simulink model "BLDC_FOC_Control_1"  (R2024b)
settings: Solver=VariableStepAuto  StartTime=0.0  StopTime=1  RelTol=1e-3
values from neighbouring files (symbols this model uses):
  iref = 70    [Parameters_List.m]
  pole_pair_number = 1    [Parameters_List.m]
  psim = 0.0175    [Parameters_List.m]
  Ts = 1e-4    (= 0.0001)    [Parameters_List.m]
  Tsc = 1e-4    (= 0.0001)    [Parameters_List.m]
  Vdc = 48    [Parameters_List.m]
libraries: fl_lib x23, nesl_utility x15, ee_lib x13, eeBldcCommutationLogic x1, eeGeneralControl x1
settings Model: Creator=subhajitroy005  LastModifiedBy=subhajitroy005

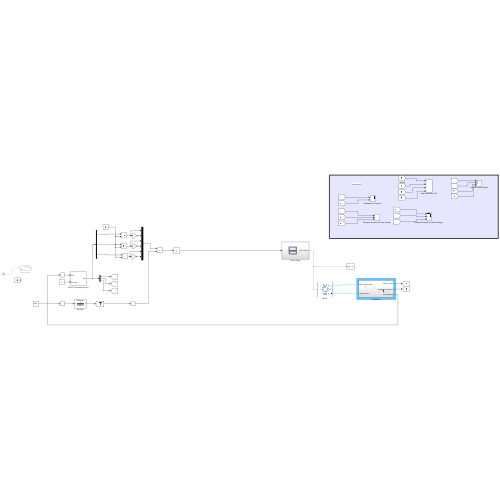
[thumbnail: Simulink's stored preview of the top-level diagram]
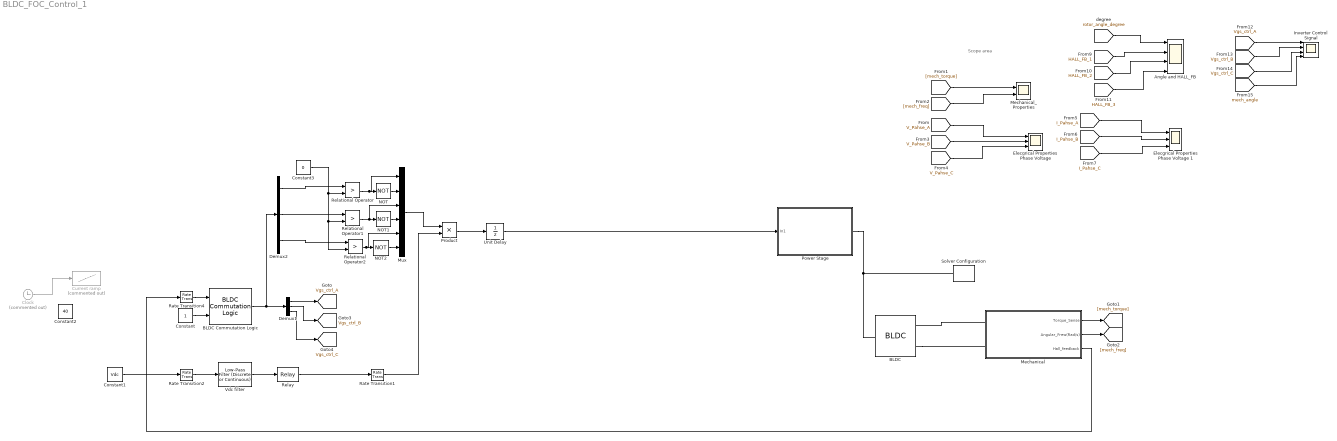
== system BLDC_FOC_Control_1 ==
  note: Scope area
  Angle and HALL_FB : Scope  NumInputPorts=4
  BLDC : ee_lib/Electromechanical/Permanent Magnet/BLDC  port_option=ee.enum.threePhasePort.composite  rotor_param=1  pm_flux_linkage=psim Wb  theta_constant=pi / (2*pole_pair_number) rad  emf_max=9.6 V  w_meas=600 rpm  DphiDtheta_tab=[0, -.1528, -.1528, .1528, .1528, 0] Wb/rad  back_emf_tab=[0, -9.6, -9.6, 9.6, 9.6, 0] V  rotor_angle_tab=[0, 7.5, 22.5, 37.5, 52.5, 60] deg  nPolePairs=pole_pair_number  axes_param=1  winding_type=ee.enum.statorconnection.wye  stator_param=2  machine_param=ee.enum.dqparameterization.constant  Ld=0.00022 H  Lq=0.00022 H  idVec=[-200, 0, 200] A  iqVec=[-200, 0, 200] A  LdMatrix=0.00022 * ones(3, 3) H  LqMatrix=0.00022 * ones(3, 3) H  L0=0.00016 H  Ls=Ls H  Lm=0 H  Ms=Ms H  Rs=Rs Ohm  zero_sequence=ee.enum.park.zerosequence.exclude  loss_param=ee.enum.ironloss.none  losses_oc=[0, 0, 0] W  losses_sc=[0, 0, 0] W  f_losses=60 Hz  Isc_losses=95 A  J=0 kg*m^2  lam=0 N*m/(rad/s)  i_d_specify=on  i_d_priority=High  i_d=0 A  i_d_nominal_specify=off  i_d_nominal_value=1  i_d_nominal_unit=A  i_q_specify=on  i_q_priority=High  i_q=0 A  i_q_nominal_specify=off  i_q_nominal_value=1  i_q_nominal_unit=A  torque_specify=off  torque_priority=None  torque=0 N*m  torque_nominal_specify=off  torque_nominal_value=1  torque_nominal_unit=N*m  angular_velocity_specify=off  angular_velocity_priority=High  angular_velocity=0 rpm  angular_velocity_nominal_specify=off  angular_velocity_nominal_value=1  angular_velocity_nominal_unit=rpm  angular_position_specify=off  angular_position_priority=High  angular_position=0 deg  angular_position_nominal_specify=off  angular_position_nominal_value=1  angular_position_nominal_unit=deg  alpha=3.93e-3 1/K  alpha_flux=-0.001 1/K  Tmeas=298.15 K  stator_thermal_mass=100 J/K  rotor_thermal_mass=200 J/K  Rm_percent_rotor=90  Rd_percent_rotor=30  temperatureA_specify=off  temperatureA_priority=High  temperatureA=25 degC  temperatureA_nominal_specify=off  temperatureA_nominal_value=1  temperatureA_nominal_unit=degC  temperatureB_specify=off  temperatureB_priority=High  temperatureB=25 degC  temperatureB_nominal_specify=off  temperatureB_nominal_value=1  temperatureB_nominal_unit=degC  temperatureC_specify=off  temperatureC_priority=High  temperatureC=25 degC  temperatureC_nominal_specify=off  temperatureC_nominal_value=1  temperatureC_nominal_unit=degC  temperatureR_specify=off  temperatureR_priority=High  temperatureR=25 degC  temperatureR_nominal_specify=off  temperatureR_nominal_value=1  temperatureR_nominal_unit=degC
      settings: InternalSimscapePortConfiguration="{\"Bottom\":[],\"Left\":[{\"id\":\"N\",\"label\":\"~\",\"type\":\"foundation.electrical.three_phase\"}],\"Right\":[{\"id\":\"R\",\"label\":\"R\",\"type\":\"foundation.mechanical.rotational.rotational\"},{\"id\":\"C\",\"label\":\"C\",\"type\":\"foundation.mechanical.rotational.rotational\"}],\"Top\":[]}"
  BLDC Commutation Logic : eeBldcCommutationLogic/BLDC Commutation Logic  Ts=Tsc
  Clock : Clock  Commented=on
  Constant : Constant
  Constant1 : Constant  Value=Vdc  VectorParams1D=off
  Constant2 : Constant  Value=40
  Constant3 : Constant  Value=0
  Current ramp : Lookup_n-D  Commented=on  NumberOfTableDimensions=1  BreakpointsForDimension1=[0 0.5 1]  Table=[0 iref iref]  InternalRulePriority=Speed  RndMeth=Simplest
  Demux1 : Demux  Outputs=3
  Demux2 : Demux  Outputs=3
  "Elecgrical Properties Phase Voltage " : Scope  NumInputPorts=3
  Elecgrical Properties Phase Voltage 1 : Scope  NumInputPorts=3
  Inverter Control Signal : Scope  NumInputPorts=4
  Mechanical : Subsystem
  Mechanical_Properties : Scope  NumInputPorts=2
  Mux : Mux  Inputs=6
  NOT : Logic  Operator=NOT  IconShape=distinctive  AllPortsSameDT=off  OutDataTypeStr=boolean
  NOT1 : Logic  Operator=NOT  IconShape=distinctive  AllPortsSameDT=off  OutDataTypeStr=boolean
  NOT2 : Logic  Operator=NOT  IconShape=distinctive  AllPortsSameDT=off  OutDataTypeStr=boolean
  Power Stage : Subsystem
  Product : Product
  Rate Transition1 : RateTransition  OutPortSampleTime=Ts
  Rate Transition2 : RateTransition  OutPortSampleTime=Tsc
  Rate Transition4 : RateTransition  OutPortSampleTime=Tsc
  Relational Operator : RelationalOperator  Operator=>  OutDataTypeStr=boolean  RndMeth=Simplest  InputSameDT=off
  Relational Operator1 : RelationalOperator  Operator=>  OutDataTypeStr=boolean  RndMeth=Simplest  InputSameDT=off
  Relational Operator2 : RelationalOperator  Operator=>  OutDataTypeStr=boolean  RndMeth=Simplest  InputSameDT=off
  Relay : Relay  OnSwitchValue=Vdc/2  OffSwitchValue=Vdc/4
  Solver Configuration : nesl_utility/Solver Configuration  PhysicalDomain=network_engine_domain  SubClassName=solver  LeftPortType=input  RightPortType=generic  Tones=[]  Harmonics=[]  SimulateNoise=off  Profile=off  UseLocalSampling=off  EnableSwitchedLinearOptims=on  FrequencyDomain=off  UseCCode=off  RelTol=0.001  AbsTol=0.001  MinStep=1e-09  ToWorkspace=off  RevertToSquareIcSolve=off  NumHomotopyIterations=100  PhasorMode=off  PhasorModeNumHarmonics=1  ConsistencySolver=NEWTON_XTOL_AFTER_FTOL  IndexReductionMethod=DerivativeReplacement  DoDC=off  ResidualTolerance=1e-09  ConsistencyTolSource=GLOBAL  ConsistencyAbsTol=0.001  ConsistencyRelTol=0.001  ConsistencyTolFactor=1e-9  UseLocalSolver=on  LocalSolverChoice=NE_BACKWARD_EULER_ADVANCER  ResolveIndetEquations=on  FunctionEvalNumThread=1  LocalSolverSampleTime=Ts  DoFixedCost=on  MaxNonlinIter=5  MaxModeIter=2  ComputeImpulses=off  ImpulseIterations=2  LinearAlgebra=auto  LinearAlgebraNumThread=0  EquationFormulation=NE_TIME_EF  DelaysMemoryBudget=1024  AutomaticFiltering=on  FilteringTimeConstant=0.001  PartitionStorageMethod=AS_NEEDED  PartitionMemoryBudget=1024  PartitionMethod=ROBUST  MultibodyUseLocalSolver=off  MultibodyLocalSolverChoice=ODE1  MultibodyLocalSolverSampleTime=0.001
  Unit Delay : UnitDelay  SampleTime=Ts  HasFrameUpgradeWarning=on
  Vdc filter : eeGeneralControl/Low-Pass Filter (Discrete or Continuous)  K=1  T=0.005  B=inf  A=-inf  init_option=Inherited from block input  x0=0  Ts=Tsc
  tag scope: Vgs_ctrl_A=global, Vgs_ctrl_B=global, Vgs_ctrl_C=global
  wires:
  Clock/1 -> Current ramp/1
  BLDC Commutation Logic/1 -> Demux1/1, Demux2/1
  Rate Transition1/1 -> Product/2
  Relay/1 -> Rate Transition1/1
  Rate Transition4/1 -> BLDC Commutation Logic/1
  Constant/1 -> BLDC Commutation Logic/2
  Rate Transition2/1 -> Vdc filter/1
  Vdc filter/1 -> Relay/1
  Product/1 -> Unit Delay/1
  Mechanical/3(Hall_feedback) -> Rate Transition4/1
  Constant1/1 -> Rate Transition2/1
  Constant3/1 -> Relational Operator2/2, Relational Operator1/2, Relational Operator/2
  Relational Operator/1 -> Mux/1, NOT/1
  Demux2/1 -> Relational Operator/1
  NOT/1 -> Mux/2
  Demux2/2 -> Relational Operator1/1
  NOT1/1 -> Mux/4
  Relational Operator1/1 -> Mux/3, NOT1/1
  Demux2/3 -> Relational Operator2/1
  Relational Operator2/1 -> Mux/5, NOT2/1
  NOT2/1 -> Mux/6
  Mux/1 -> Product/1
  Mechanical/1(Torque_Sense) -> [mech_torque]
  Mechanical/2(Angular_Frew(Rad/s)) -> [mech_freq]
  [mech_freq] -> Mechanical_Properties/2
  [mech_torque] -> Mechanical_Properties/1
  [I_Pahse_A] -> Elecgrical Properties Phase Voltage 1/1
  [I_Pahse_B] -> Elecgrical Properties Phase Voltage 1/2
  [I_Pahse_C] -> Elecgrical Properties Phase Voltage 1/3
  [V_Pahse_A] -> "Elecgrical Properties Phase Voltage "/1
  [V_Pahse_B] -> "Elecgrical Properties Phase Voltage "/2
  [V_Pahse_C] -> "Elecgrical Properties Phase Voltage "/3
  Unit Delay/1 -> Power Stage/1(In1)
  [rotor_angle_degree] -> Angle and HALL_FB/1
  [HALL_FB_1] -> Angle and HALL_FB/2
  [HALL_FB_2] -> Angle and HALL_FB/3
  [HALL_FB_3] -> Angle and HALL_FB/4
  Demux1/1 -> [Vgs_ctrl_A]
  Demux1/2 -> [Vgs_ctrl_B]
  Demux1/3 -> [Vgs_ctrl_C]
  [Vgs_ctrl_A] -> Inverter Control Signal/1
  [Vgs_ctrl_B] -> Inverter Control Signal/2
  [Vgs_ctrl_C] -> Inverter Control Signal/3
  [mech_angle] -> Inverter Control Signal/4
  connections:
  Mechanical/LConn1 -- BLDC/RConn2
  BLDC/RConn1 -- Mechanical/LConn2
  Power Stage/RConn1 -- Solver Configuration/RConn1 -- BLDC/LConn1

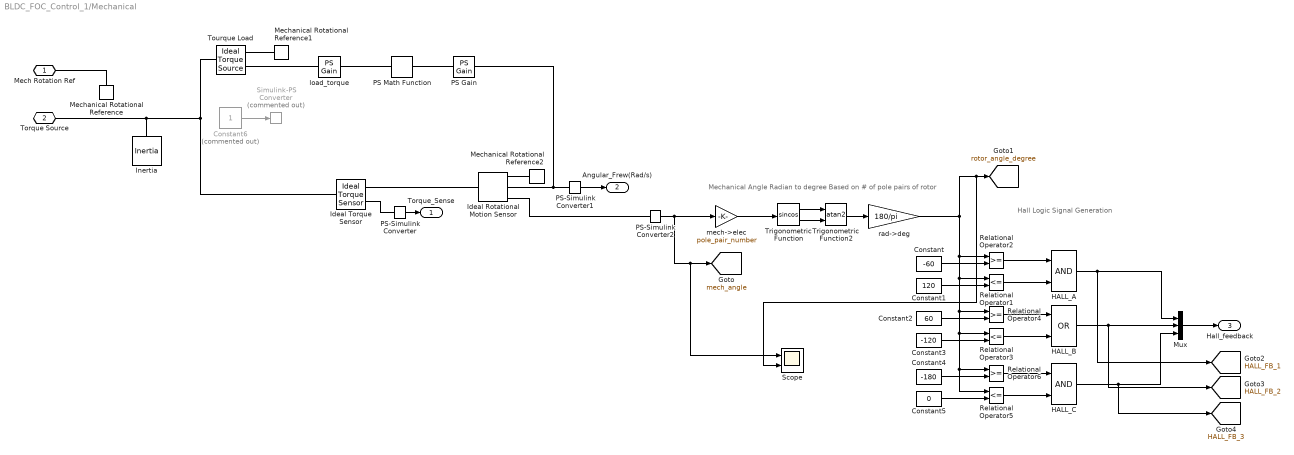
== system BLDC_FOC_Control_1/Mechanical ==
  note: Hall Logic Signal Generation
  note: Mechanical Angle Radian to degree Based on # of pole pairs of rotor
  Constant : Constant  Value=-60
  Constant1 : Constant  Value=120
  Constant2 : Constant  Value=60
  Constant3 : Constant  Value=-120
  Constant4 : Constant  Value=-180
  Constant5 : Constant  Value=0
  Constant6 : Constant  Commented=on
  HALL_A : Logic  AllPortsSameDT=off  OutDataTypeStr=boolean
  HALL_B : Logic  Operator=OR  AllPortsSameDT=off  OutDataTypeStr=boolean
  HALL_C : Logic  AllPortsSameDT=off  OutDataTypeStr=boolean
  Ideal Rotational Motion Sensor : fl_lib/Mechanical/Mechanical Sensors/Ideal Rotational Motion Sensor  reference=foundation.enum.MeasurementReference.difference  acceleration_port=false  velocity_port=true  position_port=true  wrap_angle=true  offset=0 rad
  Ideal Torque Sensor : fl_lib/Mechanical/Mechanical Sensors/Ideal Torque Sensor
  Inertia : fl_lib/Mechanical/Rotational Elements/Inertia  inertia=Jm kg*m^2  num_ports=foundation.enum.numPorts2.one  w_specify=on  w_priority=High  w=0 rad/s  w_nominal_specify=on  w_nominal_value=1  w_nominal_unit=rad/s  t_specify=off  t_priority=None  t=0 N*m  t_nominal_specify=off  t_nominal_value=1  t_nominal_unit=N*m
  Mechanical Rotational Reference : fl_lib/Mechanical/Rotational Elements/Mechanical Rotational Reference
  Mechanical Rotational Reference1 : fl_lib/Mechanical/Rotational Elements/Mechanical Rotational Reference
  Mechanical Rotational Reference2 : fl_lib/Mechanical/Rotational Elements/Mechanical Rotational Reference
  Mux : Mux  Inputs=3
  PS Gain : fl_lib/Physical Signals/Functions/PS Gain  gain=1/200 1/(rad/s)
  PS Math Function : fl_lib/Physical Signals/Functions/PS Math Function  fcn_choice=7  v=1
  PS-Simulink Converter : nesl_utility/PS-Simulink Converter  PhysicalDomain=network_engine_domain  SubClassName=ps_output  LeftPortType=input  RightPortType=output  PseudoPeriodic=off  Frequencies=[]  VectorFormat=inherit  Unit=inherit  AffineConversion=off
  PS-Simulink Converter1 : nesl_utility/PS-Simulink Converter  PhysicalDomain=network_engine_domain  SubClassName=ps_output  LeftPortType=input  RightPortType=output  PseudoPeriodic=off  Frequencies=[]  VectorFormat=inherit  Unit=inherit  AffineConversion=off
  PS-Simulink Converter2 : nesl_utility/PS-Simulink Converter  PhysicalDomain=network_engine_domain  SubClassName=ps_output  LeftPortType=input  RightPortType=output  PseudoPeriodic=off  Frequencies=[]  VectorFormat=inherit  Unit=inherit  AffineConversion=off
  Relational Operator1 : RelationalOperator  Operator=<=
  Relational Operator2 : RelationalOperator
  Relational Operator3 : RelationalOperator  Operator=<=
  Relational Operator4 : RelationalOperator
  Relational Operator5 : RelationalOperator  Operator=<=
  Relational Operator6 : RelationalOperator
  Scope : Scope  NumInputPorts=2
  Simulink-PS Converter : nesl_utility/Simulink-PS Converter  Commented=on  PhysicalDomain=network_engine_domain  SubClassName=ps_input  LeftPortType=input  RightPortType=output  PseudoPeriodic=off  Frequencies=[]  NoiseDistribution=none  NoiseParameters=[]  Unit=1  AffineConversion=off  FilteringAndDerivatives=provide  SimscapeFilterOrder=1  InputFilterTimeConstant=0.001  UdotUserProvided=0
  Tourque Load : fl_lib/Mechanical/Mechanical Sources/Ideal Torque Source
  Trigonometric Function : Trigonometry  Operator=sincos
  Trigonometric Function2 : Trigonometry  Operator=atan2
  load_torque : fl_lib/Physical Signals/Functions/PS Gain  gain=-iref*psim*pole_pair_number*1.5 N*m
  mech->elec : Gain  Gain=pole_pair_number
  rad->deg : Gain  Gain=180/pi  SaturateOnIntegerOverflow=on  OutDataTypeStr=Inherit: Same as input  ParamDataTypeStr=Inherit: Same as input
  Mech Rotation Ref : PMIOPort  Side=Left
  Torque Source : PMIOPort  Port=2  Side=Left
  Torque_Sense : Outport
  Angular_Frew(Rad/s) : Outport  Port=2
  Hall_feedback : Outport  Port=3  VectorParamsAs1DForOutWhenUnconnected=off
  tag scope: HALL_FB_1=global, HALL_FB_2=global, HALL_FB_3=global, mech_angle=global, rotor_angle_degree=global
  wires:
  PS-Simulink Converter/1 -> Torque_Sense/1
  PS-Simulink Converter1/1 -> Angular_Frew(Rad/s)/1
  Trigonometric Function2/1 -> rad->deg/1
  Trigonometric Function/1 -> Trigonometric Function2/1
  mech->elec/1 -> Trigonometric Function/1
  Trigonometric Function/2 -> Trigonometric Function2/2
  Relational Operator5/1 -> HALL_C/2
  Constant2/1 -> Relational Operator4/2
  Relational Operator1/1 -> HALL_A/2
  HALL_B/1 -> [HALL_FB_2], Mux/2
  Relational Operator3/1 -> HALL_B/2
  HALL_C/1 -> [HALL_FB_3], Mux/3
  Relational Operator6/1 -> HALL_C/1
  Constant1/1 -> Relational Operator1/2
  Constant4/1 -> Relational Operator6/2
  Constant3/1 -> Relational Operator3/2
  HALL_A/1 -> Mux/1, [HALL_FB_1]
  Constant/1 -> Relational Operator2/2
  Relational Operator4/1 -> HALL_B/1
  Relational Operator2/1 -> HALL_A/1
  Constant5/1 -> Relational Operator5/2
  Mux/1 -> Hall_feedback/1
  rad->deg/1 -> Scope/2, [rotor_angle_degree], Relational Operator4/1, Relational Operator3/1, Relational Operator5/1, Relational Operator6/1, Relational Operator1/1, Relational Operator2/1
  PS-Simulink Converter2/1 -> Scope/1, [mech_angle], mech->elec/1
  Constant6/1 -> Simulink-PS Converter/1
  connections:
  Tourque Load/LConn1 -- Ideal Torque Sensor/LConn1 -- Torque Source/RConn1 -- Inertia/LConn1
  Mech Rotation Ref/RConn1 -- Mechanical Rotational Reference/LConn1
  Tourque Load/RConn2 -- Mechanical Rotational Reference1/LConn1
  Ideal Rotational Motion Sensor/LConn1 -- Ideal Torque Sensor/RConn1
  Ideal Torque Sensor/RConn2 -- PS-Simulink Converter/LConn1
  Ideal Rotational Motion Sensor/RConn2 -- PS Gain/LConn1 -- PS-Simulink Converter1/LConn1
  Mechanical Rotational Reference2/LConn1 -- Ideal Rotational Motion Sensor/RConn1
  PS-Simulink Converter2/LConn1 -- Ideal Rotational Motion Sensor/RConn3
  PS Gain/RConn1 -- PS Math Function/LConn1
  load_torque/LConn1 -- PS Math Function/RConn1
  load_torque/RConn1 -- Tourque Load/RConn1

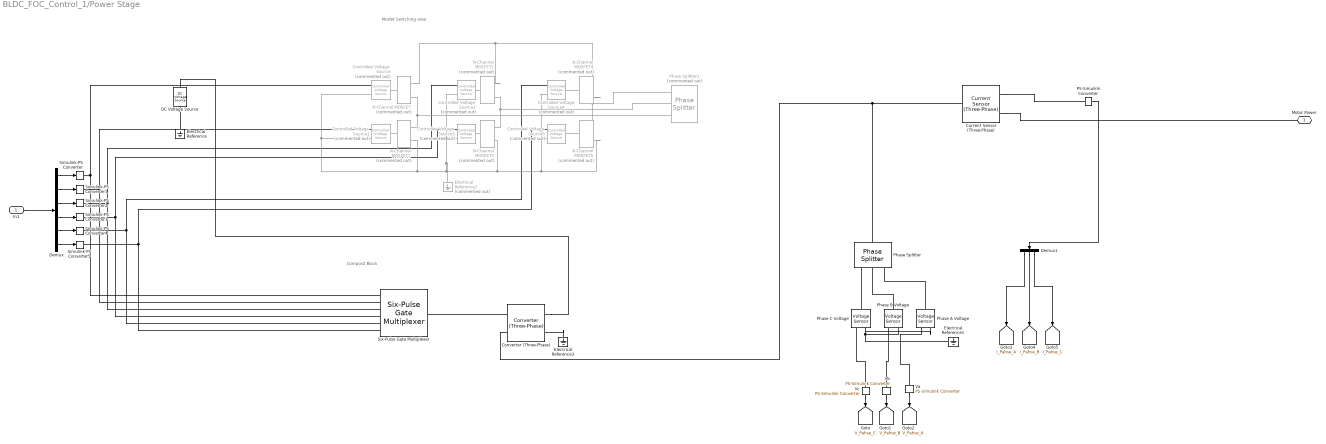
== system BLDC_FOC_Control_1/Power Stage ==
  note: Composit Block
  note: Mosfet Switching area
  In1 : Inport
  Controlled Voltage Source{,1..5} (6 alike) : fl_lib/Electrical/Electrical Sources/Controlled Voltage Source  Commented=on
  Converter (Three-Phase) : ee_lib/Semiconductors & Converters/Converters/Converter (Three-Phase)  port_option=ee.enum.threePhasePort.composite  fidelity_option=ee.enum.converters.fidelity.detailed  device_type=ee.enum.converters.switchingdevice.igbt  showThermalPort=false  K=0  Vth=0.5 V  Vgt=1 V  Vgt_off=-1 V  Ih=1 A  Vf=0.8 V  Ron=0.001 Ohm  Rds=0.001 Ohm  Goff=1e-5 1/Ohm  Eon_scalar=22.86e-3 J  Eoff_scalar=17.14e-3 J  Eoff_natural_commutation=10e-3 J  Voff=300 V  Iout_scalar=600 A  onCurrentMeasDelay=0 s  useCurrentFromPreviousCycle=false  useVoltageFromPreviousCycle=false  diode_param=ee.enum.converters.protectiondiode.nodynamics  diode_Vf=0.8 V  diode_Ron=0.001 Ohm  diode_Goff=1e-5 1/Ohm  diode_C=50 nF  diode_iRM=-235 A  diode_iF=300 A  diode_idot=-50 A/us  diode_trr_param=ee.enum.converters.diodetrr.trr_factor  diode_trr_factor=3  diode_trr=15 us  diode_Qrr=1500 s*uA  diode_rec_loss_model=ee.enum.diode.reverseRecoveryModel.fixed  diode_ErecVal=0 J  diode_scaleWithIandV=false  diode_ErecMat=zeros(2, 3) J  diode_TjrecVec=[298.15, 398.15] K  diode_IfrecVec=[.1, 1, 10] A  diode_IrecVal=10 A  diode_VrecVal=10 V  diode_tFilter=1 / 1000 / 100 s  thermal_network_parameterization=ee.enum.thermalNetworkTopology.external  Rth=[.08, .5] K/W  Rth_Cauer=[.08, .1, .5] K/W  Rth_Foster=[.08, .14, .22, .16] K/W  thermal_mass_parameterization=ee.enum.thermalNetwork.timeconstant  thermal_mass=[.01, .5] J/K  thermal_mass_Cauer=[.01, .1, .5] J/K  thermal_mass_Foster=[.001, .005, .05, .5] J/K  thermal_time_constant=[.001, .2] s  thermal_time_constant_Cauer=[.001, .1, .2] s  thermal_time_constant_Foster=[7e-05, .0007, .01, .08] s  thermal_mass_initial_temperatures=[25, 25] degC  thermal_mass_initial_temperatures_Cauer=[25, 25, 25] degC  junction_thermal_mass=0.01 J/K  Tvec_initial_Foster=[25, 25, 25, 25] degC  snubber_type=ee.enum.converters.snubber.exclude  Cs=1e-7 F  Rs=0.1 Ohm  Vce_loss=[0, 150, 300] V
  Current Sensor (Three-Phase) : ee_lib/Sensors & Transducers/Current Sensor (Three-Phase)
  DC Voltage Source : ee_lib/Additional Components/SPICE Sources/DC Voltage Source  DC=Vdc V
  Demux : Demux  Outputs=6
  Demux1 : Demux  Outputs=3
  Electrical Reference : fl_lib/Electrical/Electrical Elements/Electrical Reference
  Electrical Reference1 : fl_lib/Electrical/Electrical Elements/Electrical Reference
  Electrical Reference2 : fl_lib/Electrical/Electrical Elements/Electrical Reference  Commented=on
  Electrical Reference3 : fl_lib/Electrical/Electrical Elements/Electrical Reference
  N-Channel MOSFET{,1..5} (6 alike) : ee_lib/Semiconductors & Converters/N-Channel MOSFET  Commented=on  paramTerminal=ee.enum.mosfet.numberOfTerminals.three  parameterization=ee.enum.mosfet.parameterization.datasheet  Beta=5.0 A/V^2  Rds=0.025 Ohm  Id=6.0 A  Vgs=5 V  Vth=1.7 V  Vth0=1.7 V  lam=0 1/V  gamma_vth=0.5 V^(1/2)  phib=0.5 V  Vth1=1.9071 V  Vbs1=-1 V  Vth2=2.066 V  Vbs2=-2 V  Tmeas=25 degC  Vgs_vec=[-1, -.5, 2, 3, 4, 5] V  Vds_vec=[0, 2, 4, 8, 12, 16, 20] V  Vbs_vec=[0, -4, -6, -12] V  T_vec=[25, 125] degC  Vth_vec=[.4, 1.2, 1.4, 1.45] V  Vth_mat=[.4, .35; 1.2, 1.15; 1.4, 1.35; 1.45, 1.4] V  Ids_mat=[0, 0, 0, 0, 0, 0, 0; 0, 0, 0, 0, 0, 0, 0; 0, .003, .0038, .0043, .0046, .0048, .0049; 0, .0055, .008, .009, .0095, .01, .0101; 0, .0115, .016, .018, .019, .0195, .02; 0, .0152, .0225, .0265, .028, .0295, .03] A  Ids_mat0=[0, 0, 0, 0, 0, 0, 0; 0, 0, 0, 0, 0, 0, 0; 0, .003, .0038, .0043, .0046, .0048, .0049; 0, .0055, .008, .009, .0095, .01, .0101; 0, .0115, .016, .018, .019, .0195, .02; 0, .0152, .0225, .0265, .028, .0295, .03] A  Ids_mat_3D=zeros(6, 7, 2) A  Ids_mat_3D0=zeros(6, 7, 2) A  IV_table_symmetry=ee.enum.mosfet.symmetricNIV.no  RS=0.0001 Ohm  RD=0.01 Ohm  RB=0.001 Ohm  LeadRs=0 Ohm  LeadRd=0 Ohm  LeadRg=0 Ohm  LeadRb=0 Ohm  LS=0 nH  LD=0 nH  LG=0 nH  LB=0 nH  C_param=ee.enum.mosfet.capacitanceParam.fixedciss  C_GS=270 pF  C_GD=80 pF  C_GB=0 pF  C_DS=0 pF  C_iss=350 pF  C_rss=80 pF  C_oss=0 pF  C_iss_vec=[720, 700, 590, 470, 390, 310] pF  C_rss_vec=[450, 400, 300, 190, 95, 55] pF  C_oss_vec=[900, 810, 690, 420, 270, 170] pF  C_GS_vec=[270, 300, 290, 280, 295, 255] pF  C_GD_vec=[450, 400, 300, 190, 95, 55] pF  C_GB_vec=[270, 300, 290, 280, 295, 255] pF  C_Vgs_vec=0 V  C_DS_vec=[450, 410, 390, 230, 175, 115] pF  C_Vds_vec=[.1, .3, 1, 3, 10, 30] V  V_GS_for_cap_data=0 V  charge_linearity_param=ee.enum.mosfet.cgdLinearity.constant  C_OX=200 pF  V_C_OX=-0.5 V  charge_linearity_param_vgb=ee.enum.mosfet.cgbLinearity.instantly  charge_linearity_param_with_vgb=ee.enum.mosfet.cgbLinearityWithSeparateCgb.instantly  Di_param=ee.enum.mosfet.diodeParam.no  IsDiode=1e-12 A  Vbi=0.6 V  n=1  Cj0Diode=0 pF  TT=50e-9 s  Tmeas_dio=25 degC  TableTypeNoT=ee.enum.mosfet.tableType.IfMat  TableType=ee.enum.diode.tableType.IfMat  IfVec=[.07, .12, .19, 1.75, 4.24, 7.32, 11.2] A  IfMat=[.07, .12, .19, 1.75, 4.24, 7.32, 11.2; .16, .3, .72, 2.14, 4.02, 6.35, 9.12] A  VfVecV=[.9, 1.15, 1.25, 1.5, 1.75, 2.17, 2.6, 2.85] V  VfMatV=[.9, 1.15, 1.25, 1.5, 1.75, 2.17, 2.6, 2.85; .58, .68, .75, 1.1, 1.38, 1.77, 2.27, 2.7] V  TjVec=[25, 125] degC  VfVec=[.5, .7, .9, 1.3, 1.7, 2.1, 2.5] V  IfVecV=[.1, .2, .5, 1, 2, 4, 7, 10] A  diode_Goff=1e-12 1/Ohm  prmDatasheet=ee.enum.temperatureParameterization.none  prmEquCoeff=ee.enum.temperatureParameterization.none  dVth_dT=-6 mV/K  dVth0_dT=-6 mV/K  Rds_T2=0.037 Ohm  BEXDatasheet=-1.5  BEXEquCoeff=-1.5  etaisDatasheet=3  etaisEquCoeff=3  Tmeas2=125 degC  etaisTabulated=3  TdeviceDatasheet=25 degC  TdeviceEquCoeff=25 degC  TdeviceTabulated=25 degC  t_fault=inf s  i_g_specify=off  i_g_priority=None  i_g=0 A  i_g_nominal_specify=off  i_g_nominal_value=1  i_g_nominal_unit=A  i_d_specify=off  i_d_priority=None  i_d=0 A  i_d_nominal_specify=off  i_d_nominal_value=1  i_d_nominal_unit=A  i_b_specify=off  i_b_priority=None  i_b=0 A  i_b_nominal_specify=off  i_b_nominal_value=1  i_b_nominal_unit=A  voltage_gs_specify=off  voltage_gs_priority=None  voltage_gs=0 V  voltage_gs_nominal_specify=off  voltage_gs_nominal_value=1  voltage_gs_nominal_unit=V  voltage_ds_specify=off  voltage_ds_priority=None  voltage_ds=0 V  voltage_ds_nominal_specify=off  voltage_ds_nominal_value=1  voltage_ds_nominal_unit=V  voltage_bs_specify=off  voltage_bs_priority=None  voltage_bs=0 V  voltage_bs_nominal_specify=off  voltage_bs_nominal_value=1  voltage_bs_nominal_unit=V  v_Cgs_specify=off  v_Cgs_priority=High  v_Cgs=0 V  v_Cgs_nominal_specify=off  v_Cgs_nominal_value=1  v_Cgs_nominal_unit=V  v_Cds_specify=off  v_Cds_priority=High  v_Cds=0 V  v_Cds_nominal_specify=off  v_Cds_nominal_value=1  v_Cds_nominal_unit=V  v_Cbs_specify=off  v_Cbs_priority=High  v_Cbs=0 V  v_Cbs_nominal_specify=off  v_Cbs_nominal_value=1  v_Cbs_nominal_unit=V  thermal_network_parameterization=ee.enum.thermalNetworkTopology.junctionCase  Rth=[0, 10] K/W  Rth_Cauer=[1, 3, 10] K/W  Rth_Foster=[.08, .14, .22, .16] K/W  thermal_mass_parameterization=ee.enum.thermalNetwork.timeconstant  thermal_mass=[0, 1] J/K  thermal_mass_Cauer=[.1, .3, 1] J/K  thermal_mass_Foster=[.001, .005, .05, .5] J/K  thermal_time_constant=[0, 10] s  thermal_time_constant_Cauer=[1, 3, 10] s  thermal_time_constant_Foster=[7e-05, .0007, .01, .08] s  thermal_mass_initial_temperatures=[25, 25] degC  thermal_mass_initial_temperatures_Cauer=[25, 25, 25] degC  Tvec_initial_Foster=[25, 25, 25, 25] degC  betaref=18 A/V^2  Vfbref=-1.1 V  gamma=3.5 V^(1/2)  phib2ref=1 V  thesatref=0.4 1/V  alpha=0  Vp=5e-2 V  thesrref=0 1/V  m=8  Tref=25 degC  Rsref=2e-3 Ohm  Rdref=0.17 Ohm  Rgref=8.4 Ohm  Rbref=2e-3 Ohm  Cox=1500 pF  Cgso=100 pF  Cgdo=14 pF  Isref=5.2e-13 A  Cj0=480 pF  Tprm=1  etabet=1.3  Stvfb=5e-4 V/K  Stphib=-8.5e-4 V/K  etasat=1.04  etasr=0.65  etar=0.95  etais=3  Tsim=25 degC  Ig_specify=off  Ig_priority=None  Ig=0 A  Ig_nominal_specify=off  Ig_nominal_value=1  Ig_nominal_unit=A  Ids_specify=off  Ids_priority=None  Ids=0 A  Ids_nominal_specify=off  Ids_nominal_value=1  Ids_nominal_unit=A  Ib_specify=off  Ib_priority=None  Ib=0 A  Ib_nominal_specify=off  Ib_nominal_value=1  Ib_nominal_unit=A  V_gs_specify=off  V_gs_priority=None  V_gs=0 V  V_gs_nominal_specify=off  V_gs_nominal_value=1  V_gs_nominal_unit=V  V_ds_specify=off  V_ds_priority=None  V_ds=0 V  V_ds_nominal_specify=off  V_ds_nominal_value=1  V_ds_nominal_unit=V  V_bs_specify=off  V_bs_priority=None  V_bs=0 V  V_bs_nominal_specify=off  V_bs_nominal_value=1  V_bs_nominal_unit=V  QGoverCox_specify=off  QGoverCox_priority=None  QGoverCox=0 V  QGoverCox_nominal_specify=off  QGoverCox_nominal_value=1  QGoverCox_nominal_unit=V  QDoverCox_specify=off  QDoverCox_priority=None  QDoverCox=0 V  QDoverCox_nominal_specify=off  QDoverCox_nominal_value=1  QDoverCox_nominal_unit=V  QBoverCox_specify=off  QBoverCox_priority=None  QBoverCox=0 V  QBoverCox_nominal_specify=off  QBoverCox_nominal_value=1  QBoverCox_nominal_unit=V  T0=[25, 25] degC  T0_Cauer=[25, 25, 25] degC
  PS-Simulink Converter : nesl_utility/PS-Simulink Converter  PhysicalDomain=network_engine_domain  SubClassName=ps_output  LeftPortType=input  RightPortType=output  PseudoPeriodic=off  Frequencies=[]  VectorFormat=inherit  Unit=inherit  AffineConversion=off
  Phase A Voltage : fl_lib/Electrical/Electrical Sensors/Voltage Sensor
  Phase B Voltage : fl_lib/Electrical/Electrical Sensors/Voltage Sensor
  Phase C Voltage : fl_lib/Electrical/Electrical Sensors/Voltage Sensor
  Phase Splitter : ee_lib/Connectors & References/Phase Splitter
  Phase Splitter2 : ee_lib/Connectors & References/Phase Splitter  Commented=on
  Simulink-PS Converter{,1..5} (6 alike) : nesl_utility/Simulink-PS Converter  PhysicalDomain=network_engine_domain  SubClassName=ps_input  LeftPortType=input  RightPortType=output  PseudoPeriodic=off  Frequencies=[]  NoiseDistribution=none  NoiseParameters=[]  Unit=1  AffineConversion=off  FilteringAndDerivatives=provide  SimscapeFilterOrder=1  InputFilterTimeConstant=0.001  UdotUserProvided=0
  Six-Pulse Gate Multiplexer : ee_lib/Semiconductors & Converters/Converters/Six-Pulse Gate Multiplexer  port_option=ee.enum.controlport.ps
  Va : nesl_utility/PS-Simulink Converter  PhysicalDomain=network_engine_domain  SubClassName=ps_output  LeftPortType=input  RightPortType=output  PseudoPeriodic=off  Frequencies=[]  VectorFormat=inherit  Unit=inherit  AffineConversion=off
  Vb : nesl_utility/PS-Simulink Converter  PhysicalDomain=network_engine_domain  SubClassName=ps_output  LeftPortType=input  RightPortType=output  PseudoPeriodic=off  Frequencies=[]  VectorFormat=inherit  Unit=inherit  AffineConversion=off
  Vc : nesl_utility/PS-Simulink Converter  PhysicalDomain=network_engine_domain  SubClassName=ps_output  LeftPortType=input  RightPortType=output  PseudoPeriodic=off  Frequencies=[]  VectorFormat=inherit  Unit=inherit  AffineConversion=off
  Motor Power : PMIOPort  Side=Right
  tag scope: I_Pahse_A=global, I_Pahse_B=global, I_Pahse_C=global, V_Pahse_A=global, V_Pahse_B=global, V_Pahse_C=global
  wires:
  Demux/1 -> Simulink-PS Converter/1
  Demux/3 -> Simulink-PS Converter2/1
  Demux/2 -> Simulink-PS Converter1/1
  Demux/4 -> Simulink-PS Converter3/1
  Demux/5 -> Simulink-PS Converter4/1
  Demux/6 -> Simulink-PS Converter5/1
  PS-Simulink Converter/1 -> Demux1/1
  In1/1 -> Demux/1
  Demux1/1 -> [I_Pahse_A]
  Demux1/2 -> [I_Pahse_B]
  Demux1/3 -> [I_Pahse_C]
  Vc/1 -> [V_Pahse_C]
  Vb/1 -> [V_Pahse_B]
  Va/1 -> [V_Pahse_A]
  connections:
  Simulink-PS Converter/RConn1 -- Controlled Voltage Source/RConn1 -- Six-Pulse Gate Multiplexer/LConn1
  Simulink-PS Converter2/RConn1 -- Controlled Voltage Source2/RConn1 -- Six-Pulse Gate Multiplexer/LConn3
  Six-Pulse Gate Multiplexer/LConn2 -- Controlled Voltage Source1/RConn1 -- Simulink-PS Converter1/RConn1
  Simulink-PS Converter3/RConn1 -- Controlled Voltage Source3/RConn1 -- Six-Pulse Gate Multiplexer/LConn4
  Simulink-PS Converter4/RConn1 -- Controlled Voltage Source4/RConn1 -- Six-Pulse Gate Multiplexer/LConn5
  Simulink-PS Converter5/RConn1 -- Controlled Voltage Source5/RConn1 -- Six-Pulse Gate Multiplexer/LConn6
  Current Sensor (Three-Phase)/LConn1 -- Converter (Three-Phase)/LConn2 -- Phase Splitter/LConn1
  Phase C Voltage/LConn1 -- Phase Splitter/RConn3
  Phase B Voltage/LConn1 -- Phase Splitter/RConn2
  Phase A Voltage/LConn1 -- Phase Splitter/RConn1
  Phase A Voltage/RConn2 -- Phase C Voltage/RConn2 -- Phase B Voltage/RConn2 -- Electrical Reference1/LConn1
  Vc/LConn1 -- Phase C Voltage/RConn1
  Vb/LConn1 -- Phase B Voltage/RConn1
  Va/LConn1 -- Phase A Voltage/RConn1
  Current Sensor (Three-Phase)/RConn2 -- Motor Power/RConn1
  Current Sensor (Three-Phase)/RConn1 -- PS-Simulink Converter/LConn1
  Electrical Reference/LConn1 -- DC Voltage Source/RConn1
  N-Channel MOSFET2/RConn1 -- N-Channel MOSFET/RConn1 -- N-Channel MOSFET4/RConn1
  N-Channel MOSFET/RConn2 -- Phase Splitter2/RConn1 -- N-Channel MOSFET1/RConn1
  N-Channel MOSFET2/RConn2 -- Phase Splitter2/RConn2 -- N-Channel MOSFET3/RConn1
  N-Channel MOSFET4/RConn2 -- Phase Splitter2/RConn3 -- N-Channel MOSFET5/RConn1
  N-Channel MOSFET1/RConn2 -- Controlled Voltage Source1/RConn2 -- Controlled Voltage Source/RConn2 -- Electrical Reference2/LConn1 -- Controlled Voltage Source2/RConn2 -- Controlled Voltage Source3/RConn2 -- Controlled Voltage Source4/RConn2 -- Controlled Voltage Source5/RConn2 -- N-Channel MOSFET5/RConn2 -- N-Channel MOSFET3/RConn2
  N-Channel MOSFET/LConn1 -- Controlled Voltage Source/LConn1
  Controlled Voltage Source1/LConn1 -- N-Channel MOSFET1/LConn1
  Controlled Voltage Source2/LConn1 -- N-Channel MOSFET2/LConn1
  Controlled Voltage Source3/LConn1 -- N-Channel MOSFET3/LConn1
  Controlled Voltage Source4/LConn1 -- N-Channel MOSFET4/LConn1
  Controlled Voltage Source5/LConn1 -- N-Channel MOSFET5/LConn1
  Converter (Three-Phase)/LConn1 -- Six-Pulse Gate Multiplexer/RConn1
  Electrical Reference3/LConn1 -- Converter (Three-Phase)/RConn2
  Converter (Three-Phase)/RConn1 -- DC Voltage Source/LConn1
